simulink model "green_joint_average_motor_twin_model"  (R2023b)
settings: Solver=FixedStepDiscrete  StartTime=0.0  StopTime=GJDT_StopTime  FixedStep=GJDT_TsPlant  RelTol=1e-3
values from neighbouring files (symbols this model uses):
  GJDT_ControlMode = GJDT_ControlModeMit    [run_green_joint_average_motor_mit_step_test.m]    (also in setup_green_joint_current_loop_twin.m = GJDT_ControlModeCurrent)
  GJDT_ControlModeMit = int32(2)    [setup_green_joint_current_loop_twin.m]
  GJDT_ControlModeSpeed = int32(1)    [setup_green_joint_current_loop_twin.m]
  GJDT_IdRef_A = single(0.0)    [setup_green_joint_current_loop_twin.m]
  GJDT_IqAfter_A = single(0.3)    [run_green_joint_average_motor_twin_smoke_test.m]    (also in run_green_joint_current_loop_saturation_exit_test.m = single(1.5); setup_green_joint_current_loop_twin.m = single(1.5))
  GJDT_IqBefore_A = single(4.0)    [run_green_joint_current_loop_saturation_exit_test.m]    (also in setup_green_joint_current_loop_twin.m = single(0.0))
  GJDT_IqStepTime_s = 0.008    [run_green_joint_current_loop_saturation_exit_test.m]    (also in setup_green_joint_current_loop_twin.m = 0.001)
  GJDT_MitFfTorque_Nm = scenario.ff_torque_nm    [run_green_joint_average_motor_mit_step_test.m]    (also in setup_green_joint_current_loop_twin.m = single(0.0))
  GJDT_MitIqLimit_A = single(GJDT_ModuleConfig.defaults.torque_limit_a)    [setup_green_joint_current_loop_twin.m]
  GJDT_MitKd_NmSPerRad = single(mit_kd_nm_s_per_rad)    [setup_green_joint_current_loop_twin.m]
  GJDT_MitKp_NmPerRad = single(mit_kp_nm_per_rad)    [setup_green_joint_current_loop_twin.m]
  GJDT_MitPosAfter_Rad = scenario.pos_after_rad    [run_green_joint_average_motor_mit_step_test.m]    (also in setup_green_joint_current_loop_twin.m = single(0.20))
  GJDT_MitPosBefore_Rad = scenario.pos_before_rad    [run_green_joint_average_motor_mit_step_test.m]    (also in setup_green_joint_current_loop_twin.m = single(0.0))
  GJDT_MitPosStepTime_s = scenario.step_time_s    [run_green_joint_average_motor_mit_step_test.m]    (also in setup_green_joint_current_loop_twin.m = 0.02)
  GJDT_MitTorqueToIq_APerNm = single(1.0 /      double(GJDT_MitKtOutput_NmPerA))    [setup_green_joint_current_loop_twin.m]
  GJDT_MitVelTarget_RadS = scenario.vel_target_rad_s    [run_green_joint_average_motor_mit_step_test.m]    (also in setup_green_joint_current_loop_twin.m = single(0.0))
  GJDT_SpeedIqLimit_A = single(initial_iq_limit_a)    [design_green_joint_speed_loop.m]    (also in run_green_joint_average_motor_speed_step_test.m = scenario.iq_limit_a; setup_green_joint_current_loop_twin.m = single(4.0))
  GJDT_SpeedRefAfter_rad_s = scenario.speed_ref_after_rad_s    [run_green_joint_average_motor_speed_step_test.m]    (also in setup_green_joint_current_loop_twin.m = single(4.0))
  GJDT_SpeedRefBefore_rad_s = scenario.speed_ref_before_rad_s    [run_green_joint_average_motor_speed_step_test.m]    (also in setup_green_joint_current_loop_twin.m = single(0.0))
  GJDT_SpeedRefStepTime_s = scenario.step_time_s    [run_green_joint_average_motor_speed_step_test.m]    (also in setup_green_joint_current_loop_twin.m = 0.005)
  GJDT_Ts = 50e-6    (= 5e-05)    [setup_green_joint_current_loop_twin.m]
  GJDT_TsPlant = 5e-6    (= 5e-06)    [setup_green_joint_current_loop_twin.m]
  GJDT_TsSpeed = Ts_speed_s    [design_green_joint_speed_loop.m]    (also in setup_green_joint_current_loop_twin.m = 0.0001)
  GJDT_UseSpeedLoop = 0    [run_green_joint_average_motor_mit_step_test.m]    (also in run_green_joint_average_motor_speed_step_test.m = 1; run_green_joint_average_motor_twin_smoke_test.m; setup_green_joint_current_loop_twin.m)
  GJDT_Vbus_V = single(12.0)    [setup_green_joint_current_loop_twin.m]
  motor = evalin('base', 'motor')    [sweep_green_joint_speed_loop_100us_pll_candidates.m]
  simcfg = build_sim_config(cfg, module_1620)    [design_green_joint_current_loop_with_delay.m]
undefined symbols (not defined in the file or in its folder): inverter
libraries: mcbplantlib x1, autolibpmsmexterior x1
settings Model: DataDictionary=green_joint_average_motor_twin_interface.sldd  Creator=user  LastModifiedBy=user
settings DebuggingCC: ParameterPrecisionLossMsg=none

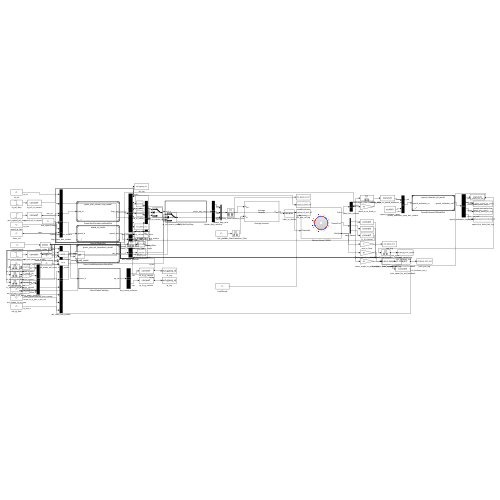
[thumbnail: Simulink's stored preview of the top-level diagram]
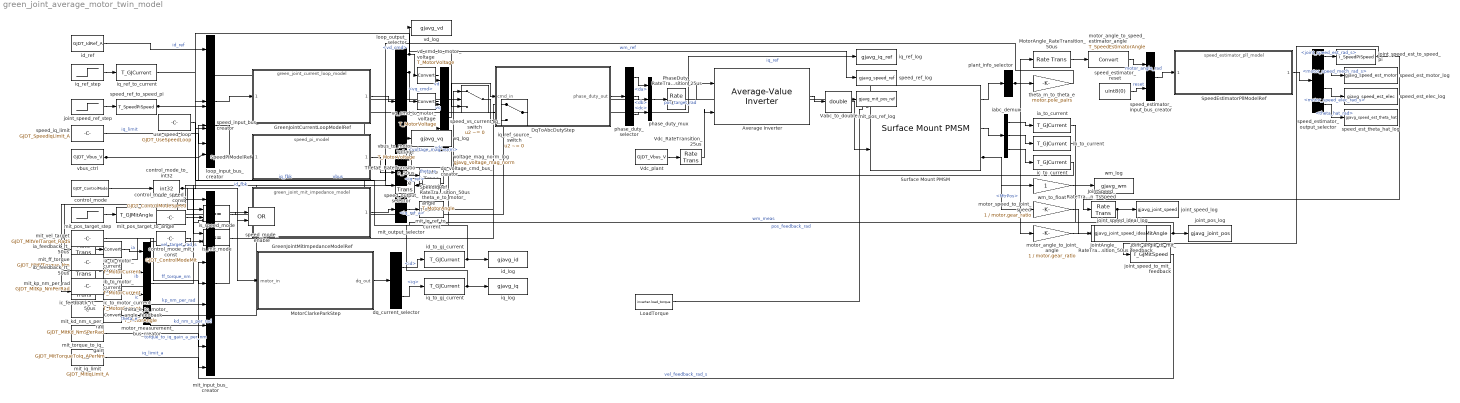
== system green_joint_average_motor_twin_model ==
  Average Inverter : mcbplantlib/Average-Value Inverter
  DqToAbcDutyStep : Subsystem  TreatAsAtomicUnit=on  RTWFcnName=DqToAbcDutyStep  RTWFileName=DqToAbcDutyStep
      settings: RTWFcnNameOpts=User specified  RTWFileNameOpts=User specified
  GreenJointCurrentLoopModelRef : ModelReference  ModelNameDialog=green_joint_current_loop_model  SimulationMode=Normal  ModelReferenceVersion=1.1
  GreenJointMitImpedanceModelRef : ModelReference  ModelNameDialog=green_joint_mit_impedance_model  SimulationMode=Normal  ModelReferenceVersion=1.1
  JointAngle_RateTransition_50us : RateTransition  OutPortSampleTime=GJDT_Ts
  JointSpeed_RateTransition_TsSpeed : RateTransition  OutPortSampleTime=GJDT_TsSpeed
  LoadTorque : Constant  Value=inverter.load_torque  OutDataTypeStr=double  SampleTime=GJDT_TsPlant
  MotorAngle_RateTransition_50us : RateTransition  OutPortSampleTime=GJDT_Ts
  MotorClarkeParkStep : Subsystem  TreatAsAtomicUnit=on  RTWFcnName=MotorClarkeParkStep  RTWFileName=MotorClarkeParkStep
      settings: RTWFcnNameOpts=User specified  RTWFileNameOpts=User specified
  PhaseDuty_RateTransition_25us : RateTransition  OutPortSampleTime=GJDT_TsPlant
  SpeedEstimatorPllModelRef : ModelReference  ModelNameDialog=speed_estimator_pll_model  SimulationMode=Normal  ModelReferenceVersion=1.1
  SpeedIqRef_RateTransition_50us : RateTransition  OutPortSampleTime=GJDT_Ts
  SpeedPiModelRef : ModelReference  ModelNameDialog=speed_pi_model  SimulationMode=Normal  ModelReferenceVersion=1.1
  Surface Mount PMSM : autolibpmsmexterior/Surface Mount PMSM  port_config=Torque  sim_type=Discrete  Ts=GJDT_TsPlant  P=motor.pole_pairs  Rs=motor.Rs  Ldq_=motor.Ld  KConstText=Permanent flux linkage constant (lambda_pm):  lambda_pm=motor.psi_f  Ke=159.9771  Kt=1.323  mechanical=[motor.J, motor.B, 0]  idq0=[0 0]  theta_init=0  omega_init=0  KConst=motor.psi_f  lambda_pm_calc=motor.psi_f  RefBlkName='autolibpmsmexterior/Surface Mount PMSM'  aMode=5  Ldq="[0.0017      0.0017]"
  ThetaE_RateTransition_50us : RateTransition  OutPortSampleTime=GJDT_Ts
  Vabc_to_double : DataTypeConversion  OutDataTypeStr=double  SaturateOnIntegerOverflow=off  RndMeth=Floor
  Vdc_RateTransition_25us : RateTransition  OutPortSampleTime=GJDT_TsPlant
  Vdc_plant : Constant  Value=GJDT_Vbus_V  OutDataTypeStr=T_GJVoltage  SampleTime=GJDT_TsPlant
  control_mode : Constant  Value=GJDT_ControlMode  OutDataTypeStr=int32  SampleTime=GJDT_Ts
  control_mode_mit_const : Constant  Value=GJDT_ControlModeMit  OutDataTypeStr=int32  SampleTime=GJDT_Ts
  control_mode_speed_const : Constant  Value=GJDT_ControlModeSpeed  OutDataTypeStr=int32  SampleTime=GJDT_Ts
  control_mode_to_int32 : DataTypeConversion  OutDataTypeStr=int32  SaturateOnIntegerOverflow=off  RndMeth=Floor
  dq_current_selector : BusSelector  OutputSignals=id,iq
  dq_voltage_cmd_bus_creator : BusCreator  Inputs=4  OutDataTypeStr=Bus: open_loop_cmd_t  NonVirtualBus=on
  ia_feedback_rt_50us : RateTransition  OutPortSampleTime=GJDT_Ts
  ia_to_current : DataTypeConversion  OutDataTypeStr=T_GJCurrent  SaturateOnIntegerOverflow=off  RndMeth=Floor
  ia_to_motor_current : DataTypeConversion  OutDataTypeStr=T_MotorCurrent  SaturateOnIntegerOverflow=off  RndMeth=Floor
  iabc_demux : Demux  Outputs=3
  ib_feedback_rt_50us : RateTransition  OutPortSampleTime=GJDT_Ts
  ib_to_current : DataTypeConversion  OutDataTypeStr=T_GJCurrent  SaturateOnIntegerOverflow=off  RndMeth=Floor
  ib_to_motor_current : DataTypeConversion  OutDataTypeStr=T_MotorCurrent  SaturateOnIntegerOverflow=off  RndMeth=Floor
  ic_feedback_rt_50us : RateTransition  OutPortSampleTime=GJDT_Ts
  ic_to_current : DataTypeConversion  OutDataTypeStr=T_GJCurrent  SaturateOnIntegerOverflow=off  RndMeth=Floor
  ic_to_motor_current : DataTypeConversion  OutDataTypeStr=T_MotorCurrent  SaturateOnIntegerOverflow=off  RndMeth=Floor
  id_log : ToWorkspace  VariableName=gjavg_id  SaveFormat=Structure With Time  SampleTime=-1
  id_ref : Constant  Value=GJDT_IdRef_A  OutDataTypeStr=T_GJCurrent  SampleTime=GJDT_Ts
  id_to_gj_current : DataTypeConversion  OutDataTypeStr=T_GJCurrent  SaturateOnIntegerOverflow=off  RndMeth=Floor
  iq_log : ToWorkspace  VariableName=gjavg_iq  SaveFormat=Structure With Time  SampleTime=-1
  iq_ref_log : ToWorkspace  VariableName=gjavg_iq_ref  SaveFormat=Structure With Time  SampleTime=-1
  iq_ref_source_switch : Switch  Criteria=u2 ~= 0  Threshold=0.5  SaturateOnIntegerOverflow=off  InputSameDT=off
  iq_ref_step : Step  Time=GJDT_IqStepTime_s  Before=GJDT_IqBefore_A  After=GJDT_IqAfter_A  SampleTime=GJDT_Ts
  iq_ref_to_current : DataTypeConversion  OutDataTypeStr=T_GJCurrent  SaturateOnIntegerOverflow=off  RndMeth=Floor
  iq_to_gj_current : DataTypeConversion  OutDataTypeStr=T_GJCurrent  SaturateOnIntegerOverflow=off  RndMeth=Floor
  is_mit_mode : RelationalOperator  Operator===  OutDataTypeStr=boolean  RndMeth=Simplest  InputSameDT=off
  is_speed_mode : RelationalOperator  Operator===  OutDataTypeStr=boolean  RndMeth=Simplest  InputSameDT=off
  joint_angle_to_mit_feedback : DataTypeConversion  OutDataTypeStr=T_GJMitAngle  SaturateOnIntegerOverflow=off  RndMeth=Floor
  joint_pos_log : ToWorkspace  VariableName=gjavg_joint_pos  SaveFormat=Structure With Time  SampleTime=-1
  joint_speed_est_to_speed_pi : DataTypeConversion  OutDataTypeStr=T_SpeedPiSpeed  SaturateOnIntegerOverflow=off  RndMeth=Floor
  joint_speed_ideal_log : ToWorkspace  VariableName=gjavg_joint_speed_ideal  SaveFormat=Structure With Time  SampleTime=-1
  joint_speed_log : ToWorkspace  VariableName=gjavg_joint_speed  SaveFormat=Structure With Time  SampleTime=-1
  joint_speed_ref_step : Step  Time=GJDT_SpeedRefStepTime_s  Before=GJDT_SpeedRefBefore_rad_s  After=GJDT_SpeedRefAfter_rad_s  SampleTime=GJDT_TsSpeed
  joint_speed_to_mit_feedback : DataTypeConversion  OutDataTypeStr=T_GJMitSpeed  SaturateOnIntegerOverflow=off  RndMeth=Floor
  loop_input_bus_creator : BusCreator  Inputs=5  OutDataTypeStr=Bus: green_joint_current_loop_input_t  NonVirtualBus=on
  loop_output_selector : BusSelector  OutputSignals=vd_cmd,vq_cmd,voltage_mag,vd_norm,vq_norm,voltage_mag_norm
  mit_ff_torque : Constant  Value=GJDT_MitFfTorque_Nm  OutDataTypeStr=T_GJMitTorque  SampleTime=GJDT_Ts
  mit_input_bus_creator : BusCreator  Inputs=9  OutDataTypeStr=Bus: green_joint_mit_input_t  NonVirtualBus=on
  mit_iq_limit : Constant  Value=GJDT_MitIqLimit_A  OutDataTypeStr=T_GJMitCurrent  SampleTime=GJDT_Ts
  mit_iq_ref_to_current : DataTypeConversion  OutDataTypeStr=T_GJCurrent  SaturateOnIntegerOverflow=off  RndMeth=Floor
  mit_kd_nm_s_per_rad : Constant  Value=GJDT_MitKd_NmSPerRad  OutDataTypeStr=T_GJMitGain  SampleTime=GJDT_Ts
  mit_kp_nm_per_rad : Constant  Value=GJDT_MitKp_NmPerRad  OutDataTypeStr=T_GJMitGain  SampleTime=GJDT_Ts
  mit_output_selector : BusSelector  OutputSignals=iq_ref_a
  mit_pos_ref_log : ToWorkspace  VariableName=gjavg_mit_pos_ref  SaveFormat=Structure With Time  SampleTime=-1
  mit_pos_target_step : Step  Time=GJDT_MitPosStepTime_s  Before=GJDT_MitPosBefore_Rad  After=GJDT_MitPosAfter_Rad  SampleTime=GJDT_Ts
  mit_pos_target_to_angle : DataTypeConversion  OutDataTypeStr=T_GJMitAngle  SaturateOnIntegerOverflow=off  RndMeth=Floor
  mit_torque_to_iq_gain : Constant  Value=GJDT_MitTorqueToIq_APerNm  OutDataTypeStr=T_GJMitGain  SampleTime=GJDT_Ts
  mit_vel_target : Constant  Value=GJDT_MitVelTarget_RadS  OutDataTypeStr=T_GJMitSpeed  SampleTime=GJDT_Ts
  motor_angle_to_joint_angle : Gain  Gain=1 / motor.gear_ratio  OutDataTypeStr=T_GJMitAngle
  motor_angle_to_speed_estimator_angle : DataTypeConversion  OutDataTypeStr=T_SpeedEstimatorAngle  SaturateOnIntegerOverflow=off  RndMeth=Floor
  motor_measurement_bus_creator : BusCreator  Inputs=4  OutDataTypeStr=Bus: motor_t  NonVirtualBus=on
  motor_speed_to_joint_speed : Gain  Gain=1 / motor.gear_ratio  OutDataTypeStr=T_SpeedPiSpeed
  phase_duty_mux : Mux  Inputs=3
  phase_duty_selector : BusSelector  OutputSignals=da,db,dc
  plant_info_selector : BusSelector  OutputSignals=MtrPos
  speed_est_elec_log : ToWorkspace  VariableName=gjavg_speed_est_elec  SaveFormat=Structure With Time  SampleTime=-1
  speed_est_motor_log : ToWorkspace  VariableName=gjavg_speed_est_motor  SaveFormat=Structure With Time  SampleTime=-1
  speed_est_theta_hat_log : ToWorkspace  VariableName=gjavg_speed_est_theta_hat  SaveFormat=Structure With Time  SampleTime=-1
  speed_estimator_input_bus_creator : BusCreator  Inputs=2  OutDataTypeStr=Bus: speed_estimator_input_t  NonVirtualBus=on
  speed_estimator_output_selector : BusSelector  OutputSignals=joint_speed_est_rad_s,motor_speed_mech_rad_s,motor_speed_elec_rad_s,theta_hat_rad
  speed_estimator_reset : Constant  Value=uint8(0)  OutDataTypeStr=T_SpeedEstimatorReset  SampleTime=GJDT_Ts
  speed_input_bus_creator : BusCreator  Inputs=3  OutDataTypeStr=Bus: speed_pi_input_t  NonVirtualBus=on
  speed_iq_limit : Constant  Value=GJDT_SpeedIqLimit_A  OutDataTypeStr=T_SpeedPiCurrent  SampleTime=GJDT_TsSpeed
  speed_mode_enable : Logic  Operator=OR  AllPortsSameDT=off  OutDataTypeStr=boolean
  speed_output_selector : BusSelector  OutputSignals=iq_ref
  speed_ref_log : ToWorkspace  VariableName=gjavg_speed_ref  SaveFormat=Structure With Time  SampleTime=-1
  speed_ref_to_speed_pi : DataTypeConversion  OutDataTypeStr=T_SpeedPiSpeed  SaturateOnIntegerOverflow=off  RndMeth=Floor
  speed_vs_current_iq_switch : Switch  Criteria=u2 ~= 0  Threshold=0.5  SaturateOnIntegerOverflow=off  InputSameDT=off
  theta_e_to_motor_angle : DataTypeConversion  OutDataTypeStr=T_MotorAngle  SaturateOnIntegerOverflow=off  RndMeth=Floor
  theta_e_to_motor_angle_feedback : DataTypeConversion  OutDataTypeStr=T_MotorAngle  SaturateOnIntegerOverflow=off  RndMeth=Floor
  theta_m_to_theta_e : Gain  Gain=motor.pole_pairs  OutDataTypeStr=T_GJFloat
  use_speed_loop : Constant  Value=GJDT_UseSpeedLoop  OutDataTypeStr=boolean  SampleTime=GJDT_Ts
  vbus_ctrl : Constant  Value=GJDT_Vbus_V  OutDataTypeStr=T_GJVoltage  SampleTime=GJDT_Ts
  vbus_to_motor_voltage : DataTypeConversion  OutDataTypeStr=T_MotorVoltage  SaturateOnIntegerOverflow=off  RndMeth=Floor
  vd_cmd_to_motor_voltage : DataTypeConversion  OutDataTypeStr=T_MotorVoltage  SaturateOnIntegerOverflow=off  RndMeth=Floor
  vd_log : ToWorkspace  VariableName=gjavg_vd  SaveFormat=Structure With Time  SampleTime=-1
  voltage_mag_norm_log : ToWorkspace  VariableName=gjavg_voltage_mag_norm  SaveFormat=Structure With Time  SampleTime=-1
  vq_cmd_to_motor_voltage : DataTypeConversion  OutDataTypeStr=T_MotorVoltage  SaturateOnIntegerOverflow=off  RndMeth=Floor
  vq_log : ToWorkspace  VariableName=gjavg_vq  SaveFormat=Structure With Time  SampleTime=-1
  wm_log : ToWorkspace  VariableName=gjavg_wm  SaveFormat=Structure With Time  SampleTime=-1
  wm_to_float : Gain  OutDataTypeStr=T_GJFloat
  wires:
  id_ref/1 -> loop_input_bus_creator/1  "id_ref"
  iq_ref_step/1 -> iq_ref_to_current/1
  joint_speed_ref_step/1 -> speed_ref_to_speed_pi/1
  speed_ref_to_speed_pi/1 -> speed_input_bus_creator/1, speed_ref_log/1  "wm_ref"
  JointSpeed_RateTransition_TsSpeed/1 -> speed_input_bus_creator/2, joint_speed_log/1  "wm_meas"
  speed_iq_limit/1 -> speed_input_bus_creator/3  "iq_limit"
  speed_input_bus_creator/1 -> SpeedPiModelRef/1
  SpeedPiModelRef/1 -> speed_output_selector/1
  speed_output_selector/1 -> SpeedIqRef_RateTransition_50us/1  "<iq_ref>"
  SpeedIqRef_RateTransition_50us/1 -> speed_vs_current_iq_switch/1
  control_mode/1 -> control_mode_to_int32/1
  control_mode_to_int32/1 -> is_speed_mode/1, is_mit_mode/1
  control_mode_speed_const/1 -> is_speed_mode/2
  control_mode_mit_const/1 -> is_mit_mode/2
  is_speed_mode/1 -> speed_mode_enable/1
  use_speed_loop/1 -> speed_mode_enable/2
  speed_mode_enable/1 -> speed_vs_current_iq_switch/2
  iq_ref_to_current/1 -> speed_vs_current_iq_switch/3
  mit_pos_target_step/1 -> mit_pos_target_to_angle/1
  mit_pos_target_to_angle/1 -> mit_input_bus_creator/1, mit_pos_ref_log/1  "pos_target_rad"
  joint_angle_to_mit_feedback/1 -> mit_input_bus_creator/2, joint_pos_log/1  "pos_feedback_rad"
  mit_vel_target/1 -> mit_input_bus_creator/3  "vel_target_rad_s"
  joint_speed_to_mit_feedback/1 -> mit_input_bus_creator/4  "vel_feedback_rad_s"
  mit_ff_torque/1 -> mit_input_bus_creator/5  "ff_torque_nm"
  mit_kp_nm_per_rad/1 -> mit_input_bus_creator/6  "kp_nm_per_rad"
  mit_kd_nm_s_per_rad/1 -> mit_input_bus_creator/7  "kd_nm_s_per_rad"
  mit_torque_to_iq_gain/1 -> mit_input_bus_creator/8  "torque_to_iq_gain_a_per_nm"
  mit_iq_limit/1 -> mit_input_bus_creator/9  "iq_limit_a"
  mit_input_bus_creator/1 -> GreenJointMitImpedanceModelRef/1
  GreenJointMitImpedanceModelRef/1 -> mit_output_selector/1
  mit_output_selector/1 -> mit_iq_ref_to_current/1  "<iq_ref_a>"
  mit_iq_ref_to_current/1 -> iq_ref_source_switch/1
  is_mit_mode/1 -> iq_ref_source_switch/2
  speed_vs_current_iq_switch/1 -> iq_ref_source_switch/3
  iq_ref_source_switch/1 -> loop_input_bus_creator/2, iq_ref_log/1  "iq_ref"
  id_to_gj_current/1 -> loop_input_bus_creator/3, id_log/1  "id_fbk"
  iq_to_gj_current/1 -> loop_input_bus_creator/4, iq_log/1  "iq_fbk"
  vbus_ctrl/1 -> loop_input_bus_creator/5, vbus_to_motor_voltage/1  "vbus"
  loop_input_bus_creator/1 -> GreenJointCurrentLoopModelRef/1
  GreenJointCurrentLoopModelRef/1 -> loop_output_selector/1
  loop_output_selector/1 -> vd_cmd_to_motor_voltage/1, vd_log/1  "<vd_cmd>"
  loop_output_selector/2 -> vq_cmd_to_motor_voltage/1, vq_log/1  "<vq_cmd>"
  ThetaE_RateTransition_50us/1 -> theta_e_to_motor_angle/1, theta_e_to_motor_angle_feedback/1
  vd_cmd_to_motor_voltage/1 -> dq_voltage_cmd_bus_creator/1  "vd"
  vq_cmd_to_motor_voltage/1 -> dq_voltage_cmd_bus_creator/2  "vq"
  theta_e_to_motor_angle/1 -> dq_voltage_cmd_bus_creator/3  "theta_e"
  vbus_to_motor_voltage/1 -> dq_voltage_cmd_bus_creator/4  "vdc"
  dq_voltage_cmd_bus_creator/1 -> DqToAbcDutyStep/1(cmd_in)
  DqToAbcDutyStep/1(phase_duty_out) -> phase_duty_selector/1
  phase_duty_selector/1 -> phase_duty_mux/1  "<da>"
  phase_duty_selector/2 -> phase_duty_mux/2  "<db>"
  phase_duty_selector/3 -> phase_duty_mux/3  "<dc>"
  phase_duty_mux/1 -> PhaseDuty_RateTransition_25us/1
  PhaseDuty_RateTransition_25us/1 -> Average Inverter/1
  Vdc_plant/1 -> Vdc_RateTransition_25us/1
  Vdc_RateTransition_25us/1 -> Average Inverter/2
  Average Inverter/1 -> Vabc_to_double/1
  Vabc_to_double/1 -> Surface Mount PMSM/2
  LoadTorque/1 -> Surface Mount PMSM/1
  Surface Mount PMSM/1 -> plant_info_selector/1
  plant_info_selector/1 -> theta_m_to_theta_e/1, motor_angle_to_joint_angle/1, MotorAngle_RateTransition_50us/1  "<MtrPos>"
  MotorAngle_RateTransition_50us/1 -> motor_angle_to_speed_estimator_angle/1
  motor_angle_to_speed_estimator_angle/1 -> speed_estimator_input_bus_creator/1  "motor_angle_rad"
  speed_estimator_reset/1 -> speed_estimator_input_bus_creator/2  "reset"
  speed_estimator_input_bus_creator/1 -> SpeedEstimatorPllModelRef/1
  SpeedEstimatorPllModelRef/1 -> speed_estimator_output_selector/1
  speed_estimator_output_selector/1 -> joint_speed_est_to_speed_pi/1  "<joint_speed_est_rad_s>"
  joint_speed_est_to_speed_pi/1 -> JointSpeed_RateTransition_TsSpeed/1, joint_speed_to_mit_feedback/1
  motor_angle_to_joint_angle/1 -> JointAngle_RateTransition_50us/1
  JointAngle_RateTransition_50us/1 -> joint_angle_to_mit_feedback/1
  theta_m_to_theta_e/1 -> ThetaE_RateTransition_50us/1
  Surface Mount PMSM/2 -> iabc_demux/1
  iabc_demux/1 -> ia_to_current/1
  iabc_demux/2 -> ib_to_current/1
  iabc_demux/3 -> ic_to_current/1
  ia_to_current/1 -> ia_feedback_rt_50us/1
  ib_to_current/1 -> ib_feedback_rt_50us/1
  ic_to_current/1 -> ic_feedback_rt_50us/1
  ia_feedback_rt_50us/1 -> ia_to_motor_current/1
  ib_feedback_rt_50us/1 -> ib_to_motor_current/1
  ic_feedback_rt_50us/1 -> ic_to_motor_current/1
  ia_to_motor_current/1 -> motor_measurement_bus_creator/1  "ia"
  ib_to_motor_current/1 -> motor_measurement_bus_creator/2  "ib"
  ic_to_motor_current/1 -> motor_measurement_bus_creator/3  "ic"
  theta_e_to_motor_angle_feedback/1 -> motor_measurement_bus_creator/4  "theta_e"
  motor_measurement_bus_creator/1 -> MotorClarkeParkStep/1(motor_in)
  MotorClarkeParkStep/1(dq_out) -> dq_current_selector/1
  dq_current_selector/1 -> id_to_gj_current/1  "<id>"
  dq_current_selector/2 -> iq_to_gj_current/1  "<iq>"
  loop_output_selector/6 -> voltage_mag_norm_log/1  "<voltage_mag_norm>"
  Surface Mount PMSM/3 -> wm_to_float/1, motor_speed_to_joint_speed/1
  wm_to_float/1 -> wm_log/1
  motor_speed_to_joint_speed/1 -> joint_speed_ideal_log/1
  speed_estimator_output_selector/2 -> speed_est_motor_log/1  "<motor_speed_mech_rad_s>"
  speed_estimator_output_selector/3 -> speed_est_elec_log/1  "<motor_speed_elec_rad_s>"
  speed_estimator_output_selector/4 -> speed_est_theta_hat_log/1  "<theta_hat_rad>"

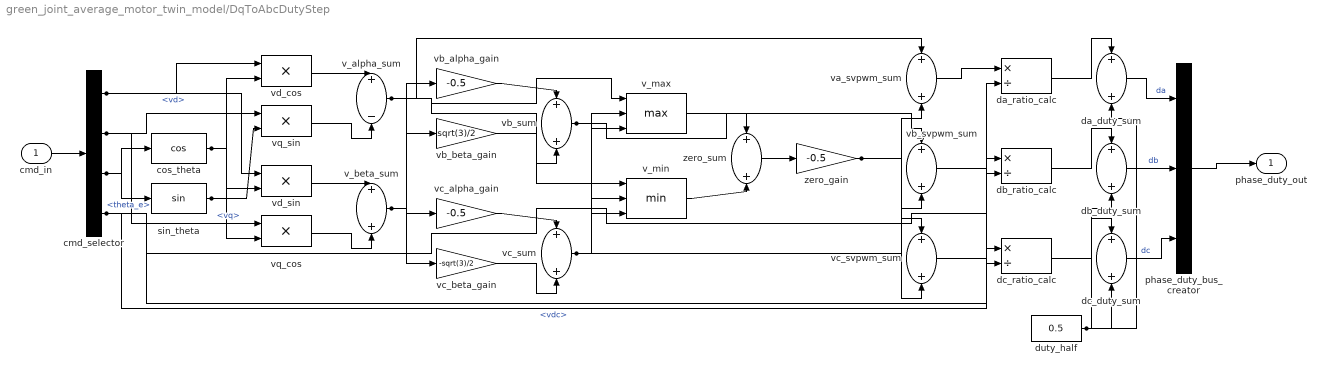
== system green_joint_average_motor_twin_model/DqToAbcDutyStep ==
  cmd_in : Inport  OutDataTypeStr=Bus: open_loop_cmd_t  BusOutputAsStruct=on
  cmd_selector : BusSelector  OutputSignals=vd,vq,theta_e,vdc
  cos_theta : Trigonometry  Operator=cos
  da_duty_sum : Sum  OutDataTypeStr=T_DutyRatio  AccumDataTypeStr=T_DutyRatio
  da_ratio_calc : Product  Inputs=*/  OutDataTypeStr=T_DutyRatio
  db_duty_sum : Sum  OutDataTypeStr=T_DutyRatio  AccumDataTypeStr=T_DutyRatio
  db_ratio_calc : Product  Inputs=*/  OutDataTypeStr=T_DutyRatio
  dc_duty_sum : Sum  OutDataTypeStr=T_DutyRatio  AccumDataTypeStr=T_DutyRatio
  dc_ratio_calc : Product  Inputs=*/  OutDataTypeStr=T_DutyRatio
  duty_half : Constant  Value=0.5  OutDataTypeStr=T_DutyRatio  SampleTime=simcfg.Ts_ctrl
  phase_duty_bus_creator : BusCreator  Inputs=3  OutDataTypeStr=Bus: phase_duty_t  NonVirtualBus=on
  sin_theta : Trigonometry
  v_alpha_sum : Sum  Inputs=+-  OutDataTypeStr=T_MotorVoltage  AccumDataTypeStr=T_MotorVoltage
  v_beta_sum : Sum  OutDataTypeStr=T_MotorVoltage  AccumDataTypeStr=T_MotorVoltage
  v_max : MinMax  Function=max  Inputs=3
  v_min : MinMax  Inputs=3
  va_svpwm_sum : Sum  OutDataTypeStr=T_MotorVoltage  AccumDataTypeStr=T_MotorVoltage
  vb_alpha_gain : Gain  Gain=-0.5  ParamDataTypeStr=T_MotorFloat  OutDataTypeStr=T_MotorVoltage
  vb_beta_gain : Gain  Gain=sqrt(3)/2  ParamDataTypeStr=T_MotorFloat  OutDataTypeStr=T_MotorVoltage
  vb_sum : Sum  OutDataTypeStr=T_MotorVoltage  AccumDataTypeStr=T_MotorVoltage
  vb_svpwm_sum : Sum  OutDataTypeStr=T_MotorVoltage  AccumDataTypeStr=T_MotorVoltage
  vc_alpha_gain : Gain  Gain=-0.5  ParamDataTypeStr=T_MotorFloat  OutDataTypeStr=T_MotorVoltage
  vc_beta_gain : Gain  Gain=-sqrt(3)/2  ParamDataTypeStr=T_MotorFloat  OutDataTypeStr=T_MotorVoltage
  vc_sum : Sum  OutDataTypeStr=T_MotorVoltage  AccumDataTypeStr=T_MotorVoltage
  vc_svpwm_sum : Sum  OutDataTypeStr=T_MotorVoltage  AccumDataTypeStr=T_MotorVoltage
  vd_cos : Product  Inputs=**  OutDataTypeStr=T_MotorVoltage
  vd_sin : Product  Inputs=**  OutDataTypeStr=T_MotorVoltage
  vq_cos : Product  Inputs=**  OutDataTypeStr=T_MotorVoltage
  vq_sin : Product  Inputs=**  OutDataTypeStr=T_MotorVoltage
  zero_gain : Gain  Gain=-0.5  ParamDataTypeStr=T_MotorFloat  OutDataTypeStr=T_MotorVoltage
  zero_sum : Sum  OutDataTypeStr=T_MotorVoltage  AccumDataTypeStr=T_MotorVoltage
  phase_duty_out : Outport  OutDataTypeStr=Bus: phase_duty_t
  wires:
  phase_duty_bus_creator/1 -> phase_duty_out/1
  dc_duty_sum/1 -> phase_duty_bus_creator/3  "dc"
  db_duty_sum/1 -> phase_duty_bus_creator/2  "db"
  da_duty_sum/1 -> phase_duty_bus_creator/1  "da"
  duty_half/1 -> dc_duty_sum/2, db_duty_sum/2, da_duty_sum/2
  dc_ratio_calc/1 -> dc_duty_sum/1
  db_ratio_calc/1 -> db_duty_sum/1
  da_ratio_calc/1 -> da_duty_sum/1
  vc_svpwm_sum/1 -> dc_ratio_calc/1
  vb_svpwm_sum/1 -> db_ratio_calc/1
  cmd_selector/4 -> dc_ratio_calc/2, db_ratio_calc/2, da_ratio_calc/2  "<vdc>"
  va_svpwm_sum/1 -> da_ratio_calc/1
  zero_gain/1 -> vc_svpwm_sum/2, vb_svpwm_sum/2, va_svpwm_sum/2
  zero_sum/1 -> zero_gain/1
  v_min/1 -> zero_sum/2
  v_max/1 -> zero_sum/1
  vc_sum/1 -> vc_svpwm_sum/1, v_min/3, v_max/3
  vb_sum/1 -> vb_svpwm_sum/1, v_min/2, v_max/2
  vc_beta_gain/1 -> vc_sum/2
  vc_alpha_gain/1 -> vc_sum/1
  vb_beta_gain/1 -> vb_sum/2
  vb_alpha_gain/1 -> vb_sum/1
  v_beta_sum/1 -> vc_beta_gain/1, vb_beta_gain/1
  v_alpha_sum/1 -> va_svpwm_sum/1, v_min/1, v_max/1, vc_alpha_gain/1, vb_alpha_gain/1
  vq_cos/1 -> v_beta_sum/2
  vd_sin/1 -> v_beta_sum/1
  vq_sin/1 -> v_alpha_sum/2
  vd_cos/1 -> v_alpha_sum/1
  sin_theta/1 -> vd_sin/2, vq_sin/2
  cmd_selector/2 -> vq_cos/1, vq_sin/1  "<vq>"
  cos_theta/1 -> vq_cos/2, vd_cos/2
  cmd_selector/1 -> vd_sin/1, vd_cos/1  "<vd>"
  cmd_selector/3 -> sin_theta/1, cos_theta/1  "<theta_e>"
  cmd_in/1 -> cmd_selector/1

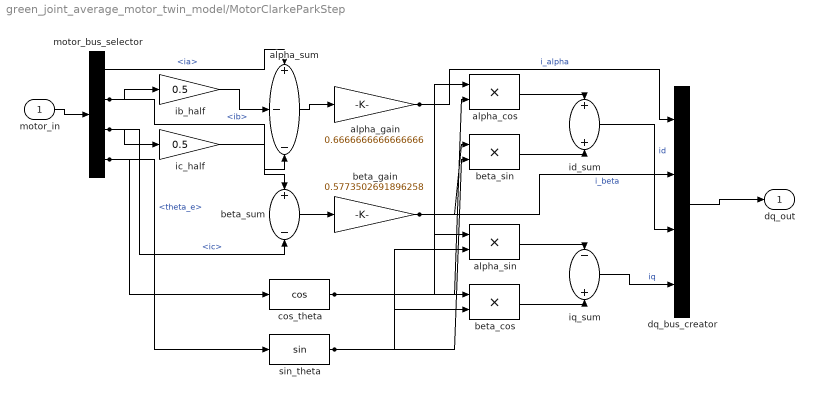
== system green_joint_average_motor_twin_model/MotorClarkeParkStep ==
  motor_in : Inport  OutDataTypeStr=Bus: motor_t  BusOutputAsStruct=on
  alpha_cos : Product  Inputs=**  OutDataTypeStr=T_MotorCurrent  SaturateOnIntegerOverflow=on
  alpha_gain : Gain  Gain=0.6666666666666666  ParamDataTypeStr=T_MotorCurrent  OutDataTypeStr=T_MotorCurrent  SaturateOnIntegerOverflow=on
  alpha_sin : Product  Inputs=**  OutDataTypeStr=T_MotorCurrent  SaturateOnIntegerOverflow=on
  alpha_sum : Sum  Inputs=+--  OutDataTypeStr=T_MotorCurrent  AccumDataTypeStr=T_MotorCurrent  SaturateOnIntegerOverflow=on
  beta_cos : Product  Inputs=**  OutDataTypeStr=T_MotorCurrent  SaturateOnIntegerOverflow=on
  beta_gain : Gain  Gain=0.5773502691896258  ParamDataTypeStr=T_MotorCurrent  OutDataTypeStr=T_MotorCurrent  SaturateOnIntegerOverflow=on
  beta_sin : Product  Inputs=**  OutDataTypeStr=T_MotorCurrent  SaturateOnIntegerOverflow=on
  beta_sum : Sum  Inputs=+-  OutDataTypeStr=T_MotorCurrent  AccumDataTypeStr=T_MotorCurrent  SaturateOnIntegerOverflow=on
  cos_theta : Trigonometry  Operator=cos
  dq_bus_creator : BusCreator  Inputs=4  OutDataTypeStr=Bus: motor_dq_t  NonVirtualBus=on
  ib_half : Gain  Gain=0.5  ParamDataTypeStr=T_MotorCurrent  OutDataTypeStr=T_MotorCurrent  SaturateOnIntegerOverflow=on
  ic_half : Gain  Gain=0.5  ParamDataTypeStr=T_MotorCurrent  OutDataTypeStr=T_MotorCurrent  SaturateOnIntegerOverflow=on
  id_sum : Sum  OutDataTypeStr=T_MotorCurrent  AccumDataTypeStr=T_MotorCurrent  SaturateOnIntegerOverflow=on
  iq_sum : Sum  Inputs=-+  OutDataTypeStr=T_MotorCurrent  AccumDataTypeStr=T_MotorCurrent  SaturateOnIntegerOverflow=on
  motor_bus_selector : BusSelector  OutputSignals=ia,ib,ic,theta_e
  sin_theta : Trigonometry
  dq_out : Outport  OutDataTypeStr=Bus: motor_dq_t
  wires:
  dq_bus_creator/1 -> dq_out/1
  iq_sum/1 -> dq_bus_creator/4  "iq"
  id_sum/1 -> dq_bus_creator/3  "id"
  beta_cos/1 -> iq_sum/2
  alpha_sin/1 -> iq_sum/1
  beta_sin/1 -> id_sum/2
  alpha_cos/1 -> id_sum/1
  sin_theta/1 -> alpha_sin/2, beta_sin/2
  beta_gain/1 -> dq_bus_creator/2, beta_cos/1, beta_sin/1  "i_beta"
  cos_theta/1 -> beta_cos/2, alpha_cos/2
  alpha_gain/1 -> dq_bus_creator/1, alpha_sin/1, alpha_cos/1  "i_alpha"
  motor_bus_selector/4 -> sin_theta/1, cos_theta/1  "<theta_e>"
  beta_sum/1 -> beta_gain/1
  alpha_sum/1 -> alpha_gain/1
  ic_half/1 -> alpha_sum/3
  ib_half/1 -> alpha_sum/2
  motor_bus_selector/3 -> beta_sum/2, ic_half/1  "<ic>"
  motor_bus_selector/2 -> beta_sum/1, ib_half/1  "<ib>"
  motor_bus_selector/1 -> alpha_sum/1  "<ia>"
  motor_in/1 -> motor_bus_selector/1
